simulink model "proj"  (R2018b)
settings: Solver=ode4  StartTime=0.0  StopTime=200  FixedStep=0.05  RelTol=1e-3  EnableMultiTasking=on
settings Model: Creator=Student  LastModifiedBy=gosci
settings DataIOCC: LimitDataPoints=on  SaveFormat=Array
settings OptimizationCC: LifeSpan=inf
settings DebuggingCC: SolverPrmCheckMsg=warning  SFUnexpectedBacktrackingDiag=warning  SFNoUnconditionalDefaultTransitionDiag=warning  SFExecutionAtInitializationDiag=none
settings HardwareCC: ProdBitPerPointer=32  ProdBitPerSizeT=32  ProdBitPerPtrDiffT=32  ProdLargestAtomicFloat=None  ProdIntDivRoundTo=Undefined  ProdEndianess=Unspecified  ProdWordSize=32  ProdHWDeviceType=32-bit Generic
settings ModelReferenceCC: PropagateSignalLabelsOutOfModel=off
settings SFSimCC: SimUseLocalCustomCode=off
settings RTWCC: RTWUseLocalCustomCode=off
settings CodeAppCC: StateflowObjectComments=on
settings GRTTargetCC: TargetLangStandard=C89/C90 (ANSI)  GeneratePreprocessorConditionals=Disable all
settings ConfigComp: CovMetricSettings=dw  CovHtmlReporting=on  CovSaveCumulativeToWorkspaceVar=on  CovSaveSingleToWorkspaceVar=on  CovExternalEMLEnable=off  CovSFcnEnable=off

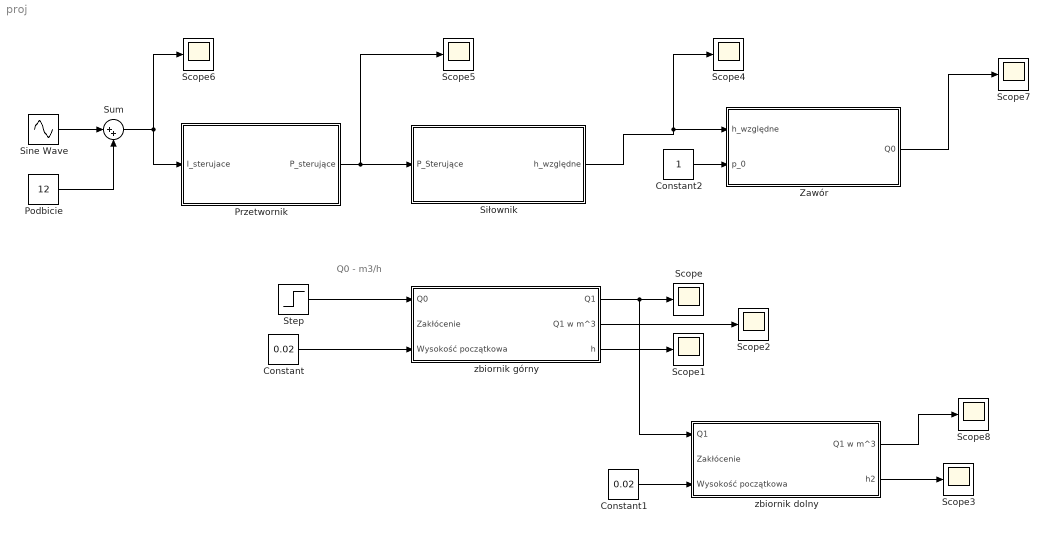
== system proj ==
  note: Q0 - m3/h
  Constant : Constant  Value=0.02
  Constant1 : Constant  Value=0.02
  Constant2 : Constant
  Podbicie : Constant  Value=12
  Przetwornik : Subsystem
  Scope{,1..8} (9 alike) : Scope
  Sine Wave : Sin  Amplitude=8  Frequency=1/20  SampleTime=0
  "Siłownik " : Subsystem
  Step : Step  Time=10  After=6  SampleTime=0
  Sum : Sum  Inputs=|++
  Zawór : Subsystem
  zbiornik dolny : Subsystem
  zbiornik górny : Subsystem
  wires:
  Step/1 -> zbiornik górny/1(Q0)
  Constant/1 -> zbiornik górny/3("Wysokość początkowa ")
  zbiornik górny/3("h ") -> Scope1/1
  zbiornik górny/2("Q1 w m^3 ") -> Scope2/1
  zbiornik górny/1(Q1) -> zbiornik dolny/1("Q1 "), Scope/1
  Constant1/1 -> zbiornik dolny/3("Wysokość początkowa ")
  zbiornik dolny/2("h2 ") -> Scope3/1
  Przetwornik/1("P_sterujące ") -> Scope5/1, "Siłownik "/1(P_Sterujące)
  "Siłownik "/1("h_względne ") -> Zawór/1(h_względne), Scope4/1
  Podbicie/1 -> Sum/2
  Sine Wave/1 -> Sum/1
  Sum/1 -> Scope6/1, Przetwornik/1(I_sterujace)
  Constant2/1 -> Zawór/2(p_0)
  Zawór/1(Q0) -> Scope7/1
  zbiornik dolny/1("Q1 w m^3 ") -> Scope8/1

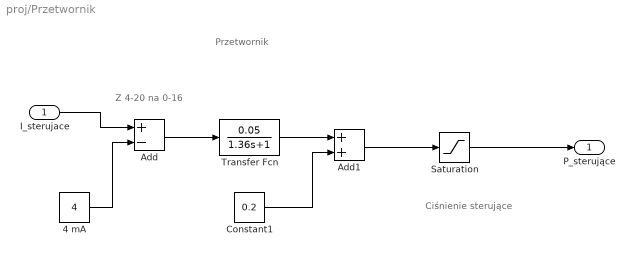
== system proj/Przetwornik ==
  note: Ciśnienie sterujące
  note: Przetwornik
  note: Z 4-20 na 0-16
  I_sterujace : Inport
  4 mA : Constant  Value=4
  Add : Sum  Inputs=+-
  Add1 : Sum
  Constant1 : Constant  Value=0.2
  Saturation : Saturate  UpperLimit=1  LowerLimit=0.2
  Transfer Fcn : TransferFcn  Numerator=[0.05]  Denominator=[1.36 1]
  "P_sterujące " : Outport
  wires:
  I_sterujace/1 -> Add/1
  Add/1 -> Transfer Fcn/1
  Transfer Fcn/1 -> Add1/1
  4 mA/1 -> Add/2
  Constant1/1 -> Add1/2
  Add1/1 -> Saturation/1
  Saturation/1 -> "P_sterujące "/1

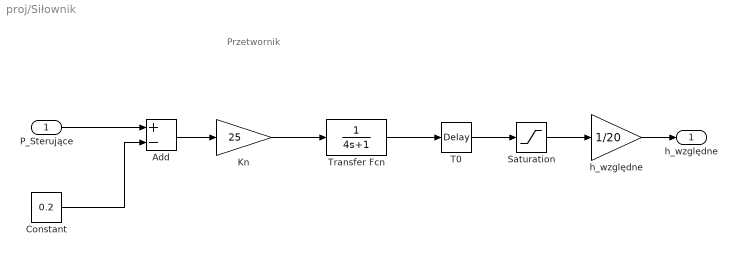
== system proj/Siłownik  ==
  note: Przetwornik
  P_Sterujące : Inport
  Add : Sum  Inputs=+-
  Constant : Constant  Value=0.2
  Kn : Gain  Gain=25
  Saturation : Saturate  UpperLimit=20  LowerLimit=0
  T0 : TransportDelay  DelayTime=1.5
  Transfer Fcn : TransferFcn  Denominator=[4 1]
  h_względne : Gain  Gain=1/20
  "h_względne " : Outport
  wires:
  P_Sterujące/1 -> Add/1
  Transfer Fcn/1 -> T0/1
  Constant/1 -> Add/2
  T0/1 -> Saturation/1
  Add/1 -> Kn/1
  Kn/1 -> Transfer Fcn/1
  h_względne/1 -> "h_względne "/1
  Saturation/1 -> h_względne/1

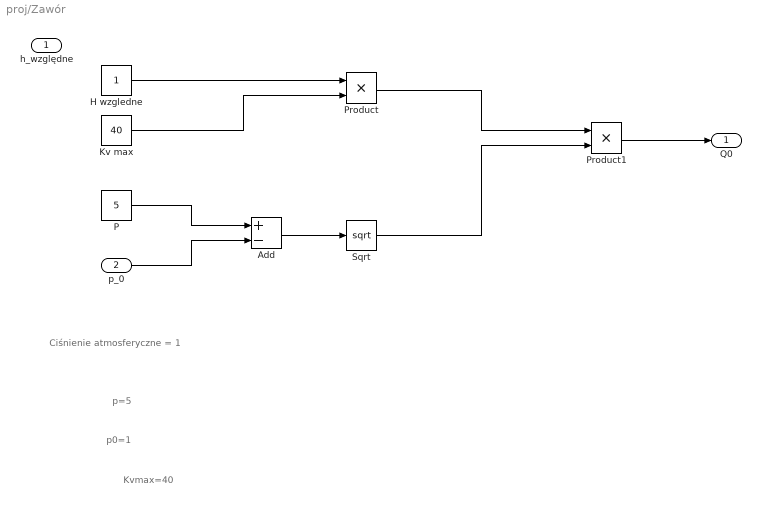
== system proj/Zawór ==
  note: Kvmax=40
  note: p0=1
  note: p=5
  note: Ciśnienie atmosferyczne = 1
  h_względne : Inport
  p_0 : Inport  Port=2
  Add : Sum  Inputs=+-
  H wzgledne : Constant
  Kv max : Constant  Value=40
  P : Constant  Value=5
  Product : Product
  Product1 : Product
  Sqrt : Sqrt  SaturateOnIntegerOverflow=on
  Q0 : Outport
  wires:
  P/1 -> Add/1
  p_0/1 -> Add/2
  Kv max/1 -> Product/2
  Add/1 -> Sqrt/1
  Sqrt/1 -> Product1/2
  Product1/1 -> Q0/1
  Product/1 -> Product1/1
  H wzgledne/1 -> Product/1

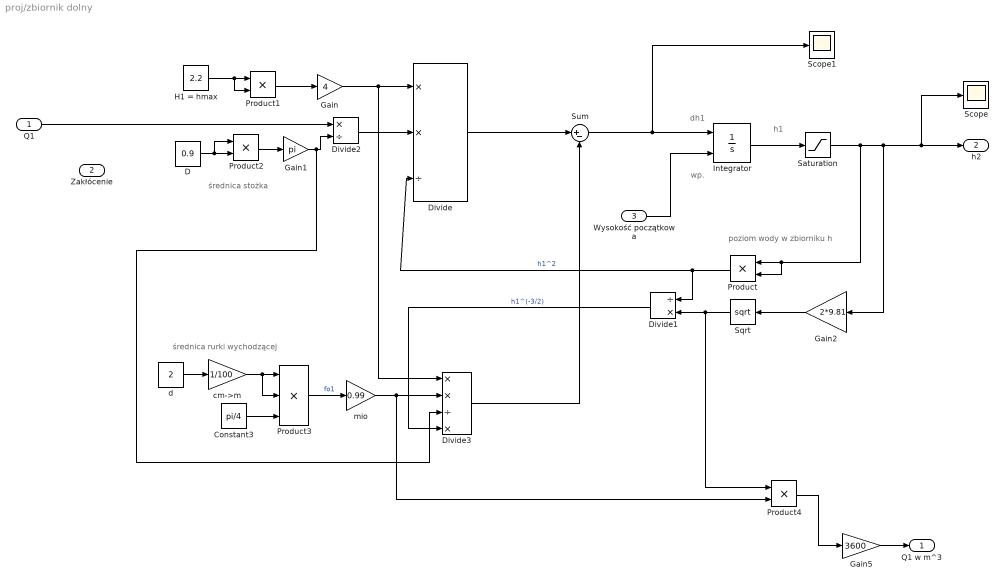
== system proj/zbiornik dolny ==
  note: poziom wody w zbiorniku h
  note: średnica stożka
  note: średnica rurki wychodzącej
  note: wp.
  note: h1
  note: dh1
  "Q1 " : Inport
  "Zakłócenie " : Inport  Port=2
  "Wysokość początkowa " : Inport  Port=3
  Constant3 : Constant  Value=pi/4
  D : Constant  Value=0.9
  Divide : Product  Inputs=**/  SaturateOnIntegerOverflow=on  RndMeth=Zero
  Divide1 : Product  Inputs=/*
  Divide2 : Product  Inputs=*/
  Divide3 : Product  Inputs=**/*
  Gain : Gain  Gain=4
  Gain1 : Gain  Gain=pi
  Gain2 : Gain  Gain=2*9.81
  Gain5 : Gain  Gain=3600
  H1 = hmax : Constant  Value=2.2
  Integrator : Integrator  InitialConditionSource=external
  Product{,1..2,4} (4 alike) : Product
  Product3 : Product  Inputs=3
  Saturation : Saturate  UpperLimit=2.1  LowerLimit=0.01
  Scope : Scope
  Scope1 : Scope
  Sqrt : Sqrt  SaturateOnIntegerOverflow=on
  Sum : Sum  Inputs=|+-
  "cm->m " : Gain  Gain=1/100
  "d " : Constant  Value=2
  mio : Gain  Gain=0.99
  "Q1 w m^3 " : Outport
  "h2 " : Outport  Port=2
  wires:
  "Wysokość początkowa "/1 -> Integrator/2
  Gain2/1 -> Sqrt/1
  Integrator/1 -> Saturation/1
  Product1/1 -> Gain/1
  H1 = hmax/1 -> Product1/2, Product1/1
  Gain1/1 -> Divide3/3, Divide2/2
  Divide2/1 -> Divide/2
  Product2/1 -> Gain1/1
  D/1 -> Product2/1, Product2/2
  Gain/1 -> Divide/1, Divide3/1
  Product/1 -> Divide1/1, Divide/3  "h1^2"
  Divide/1 -> Sum/1
  Constant3/1 -> Product3/3
  "d "/1 -> "cm->m "/1
  Product3/1 -> mio/1  "fo1"
  Divide1/1 -> Divide3/4  "h1^(-3/2)"
  mio/1 -> Product4/2, Divide3/2
  Divide3/1 -> Sum/2
  "Q1 "/1 -> Divide2/1
  Saturation/1 -> Scope/1, "h2 "/1, Gain2/1, Product/1, Product/2
  "cm->m "/1 -> Product3/1, Product3/2
  Sum/1 -> Integrator/1, Scope1/1
  Sqrt/1 -> Product4/1, Divide1/2
  Product4/1 -> Gain5/1
  Gain5/1 -> "Q1 w m^3 "/1

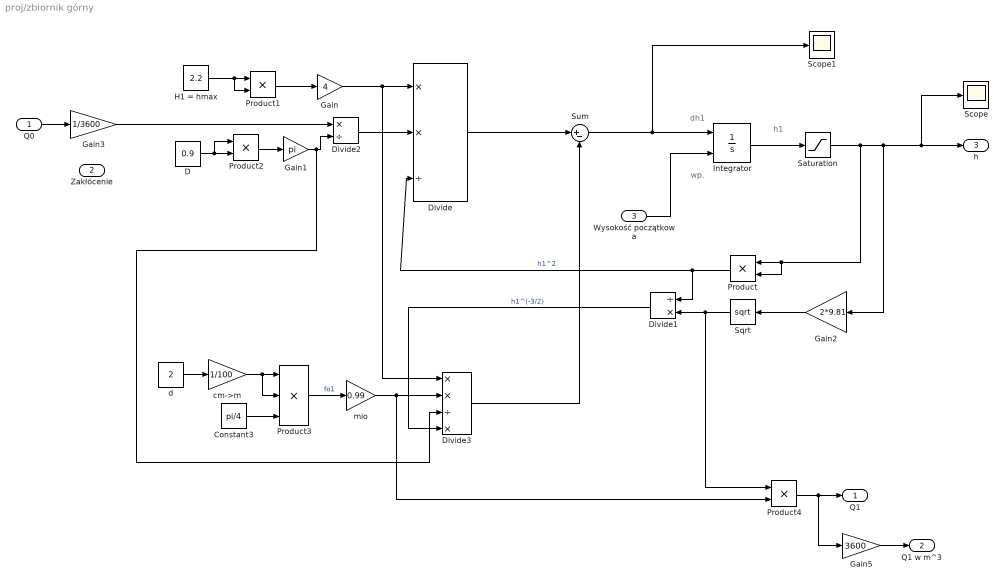
== system proj/zbiornik górny ==
  note: wp.
  note: h1
  note: dh1
  Q0 : Inport
  "Zakłócenie " : Inport  Port=2
  "Wysokość początkowa " : Inport  Port=3
  Constant3 : Constant  Value=pi/4
  D : Constant  Value=0.9
  Divide : Product  Inputs=**/  SaturateOnIntegerOverflow=on  RndMeth=Zero
  Divide1 : Product  Inputs=/*
  Divide2 : Product  Inputs=*/
  Divide3 : Product  Inputs=**/*
  Gain : Gain  Gain=4
  Gain1 : Gain  Gain=pi
  Gain2 : Gain  Gain=2*9.81
  Gain3 : Gain  Gain=1/3600
  Gain5 : Gain  Gain=3600
  H1 = hmax : Constant  Value=2.2
  Integrator : Integrator  InitialConditionSource=external
  Product{,1..2,4} (4 alike) : Product
  Product3 : Product  Inputs=3
  Saturation : Saturate  UpperLimit=2.1  LowerLimit=0.01
  Scope : Scope
  Scope1 : Scope
  Sqrt : Sqrt  SaturateOnIntegerOverflow=on
  Sum : Sum  Inputs=|+-
  "cm->m " : Gain  Gain=1/100
  "d " : Constant  Value=2
  mio : Gain  Gain=0.99
  Q1 : Outport
  "Q1 w m^3 " : Outport  Port=2
  "h " : Outport  Port=3
  wires:
  "Wysokość początkowa "/1 -> Integrator/2
  Gain2/1 -> Sqrt/1
  Integrator/1 -> Saturation/1
  Product1/1 -> Gain/1
  H1 = hmax/1 -> Product1/2, Product1/1
  Gain1/1 -> Divide3/3, Divide2/2
  Divide2/1 -> Divide/2
  Product2/1 -> Gain1/1
  D/1 -> Product2/1, Product2/2
  Gain/1 -> Divide3/1, Divide/1
  Product/1 -> Divide1/1, Divide/3  "h1^2"
  Divide/1 -> Sum/1
  Constant3/1 -> Product3/3
  "d "/1 -> "cm->m "/1
  Product3/1 -> mio/1  "fo1"
  Divide1/1 -> Divide3/4  "h1^(-3/2)"
  mio/1 -> Product4/2, Divide3/2
  Divide3/1 -> Sum/2
  Gain3/1 -> Divide2/1
  Saturation/1 -> Scope/1, "h "/1, Gain2/1, Product/1, Product/2
  "cm->m "/1 -> Product3/1, Product3/2
  Sum/1 -> Integrator/1, Scope1/1
  Q0/1 -> Gain3/1
  Sqrt/1 -> Product4/1, Divide1/2
  Product4/1 -> Gain5/1, Q1/1
  Gain5/1 -> "Q1 w m^3 "/1
